simulink model "ProdSystem_BaseStockAssumptionsAndCosts"  (R2015a)
settings: Solver=ode45  SolverMode=SingleTasking  StartTime=0  StopTime=100000000  RelTol=1e-3
libraries: simeventslib x10, simulink x1
settings Model: CovSFcnEnable=off  Creator=AnotherUser  LastModifiedBy=gthiers3
settings OptimizationCC: BlockReduction=off  BooleanDataType=off
settings DebuggingCC: SaveWithParameterizedLinksMsg=none  UnderspecifiedInitializationDetection=Classic  MergeDetectMultiDrivingBlocksExec=none  SignalResolutionControl=TryResolveAllWithWarning
settings HardwareCC: TargetUnknown=on

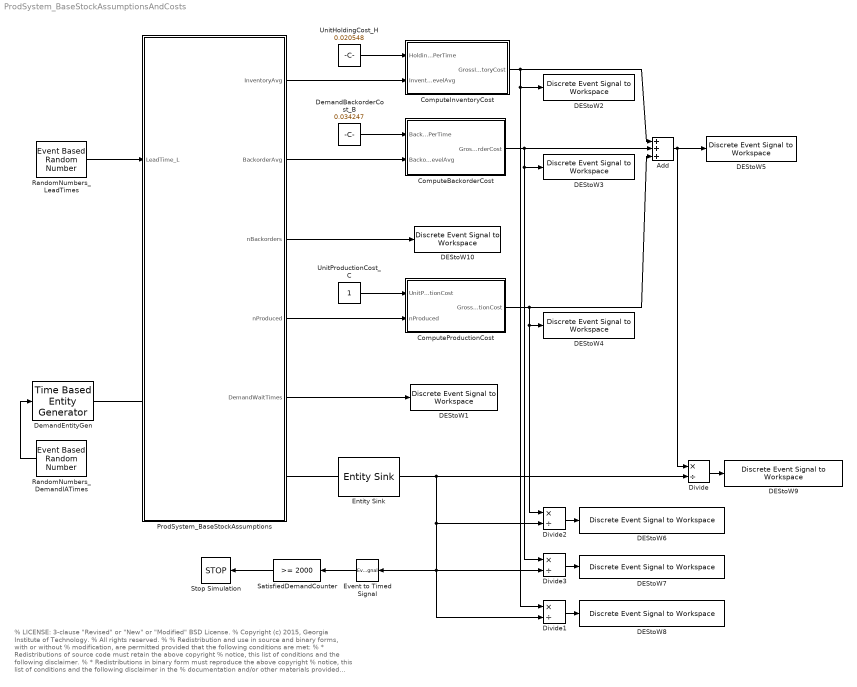
== system ProdSystem_BaseStockAssumptionsAndCosts ==
  note: % LICENSE: 3-clause "Revised" or "New" or "Modified" BSD License.
      | % Copyright (c) 2015, Georgia Institute of Technology.
      | % All rights reserved.
      | %
      | % Redistribution and use in source and binary forms, with or without
      | % modification, are permitted provided that the following conditions are met:
      | % * Redistributions of source code must retain the above copyright
      | % notice, this list of conditions and the following disclaimer.
      | % * Redistributions in binary form must reproduce the above copyright
      | % notice, this list of conditions and the following disclaimer in the
      | % documentation and/or other materials provided with the distribution.
      | % * Neither the name of the Georgia Institute of Technology nor the
      | % names of its contributors may be used to endorse or promote products
      | % derived from this software without specific prior written permission.
      | %
      | % THIS SOFTWARE IS PROVIDED BY THE COPYRIGHT HOLDERS AND CONTRIBUTORS "AS IS" AND
      | % ANY EXPRESS OR IMPLIED WARRANTIES, INCLUDING, BUT NOT LIMITED TO, THE IMPLIED
      | % WARRANTIES OF MERCHANTABILITY AND FITNESS FOR A PARTICULAR PURPOSE ARE
      | % DISCLAIMED. IN NO EVENT SHALL THE GEORGIA INSTITUTE OF TECHNOLOGY BE LIABLE FOR
      | % ANY DIRECT, INDIRECT, INCIDENTAL, SPECIAL, EXEMPLARY, OR CONSEQUENTIAL DAMAGES
      | % (INCLUDING, BUT NOT LIMITED TO, PROCUREMENT OF SUBSTITUTE GOODS OR SERVICES;
      | % LOSS OF USE, DATA, OR PROFITS; OR BUSINESS INTERRUPTION) HOWEVER CAUSED AND
      | % ON ANY THEORY OF LIABILITY, WHETHER IN CONTRACT, STRICT LIABILITY, OR TORT
      | % (INCLUDING NEGLIGENCE OR OTHERWISE) ARISING IN ANY WAY OUT OF THE USE OF THIS
      | % SOFTWARE, EVEN IF ADVISED OF THE POSSIBILITY OF SUCH DAMAGE.
  Add : Sum  Inputs=+++
  ComputeBackorderCost : Subsystem
  ComputeInventoryCost : Subsystem
  ComputeProductionCost : Subsystem
  DEStoW1 : simeventslib/SimEvents Sinks/Discrete Event Signal to Workspace  VariableName=DemandWaitTimes  SaveFormat=Structure With Time  isMonitorOnly=off  isRecordIC=off
  DEStoW10 : simeventslib/SimEvents Sinks/Discrete Event Signal to Workspace  VariableName=nBackorders  SaveFormat=Structure With Time  isMonitorOnly=off  isRecordIC=off
  DEStoW2 : simeventslib/SimEvents Sinks/Discrete Event Signal to Workspace  VariableName=GrossInventoryCost  SaveFormat=Structure With Time  isMonitorOnly=off  isRecordIC=off
  DEStoW3 : simeventslib/SimEvents Sinks/Discrete Event Signal to Workspace  VariableName=GrossBackorderCost  SaveFormat=Structure With Time  isMonitorOnly=off  isRecordIC=off
  DEStoW4 : simeventslib/SimEvents Sinks/Discrete Event Signal to Workspace  VariableName=GrossProductionCost  SaveFormat=Structure With Time  isMonitorOnly=off  isRecordIC=off
  DEStoW5 : simeventslib/SimEvents Sinks/Discrete Event Signal to Workspace  VariableName=GrossCost  SaveFormat=Structure With Time  isMonitorOnly=off  isRecordIC=off
  DEStoW6 : simeventslib/SimEvents Sinks/Discrete Event Signal to Workspace  VariableName=GrossProductionCost_PerSatDmd  SaveFormat=Structure With Time  isMonitorOnly=off  isRecordIC=off
  DEStoW7 : simeventslib/SimEvents Sinks/Discrete Event Signal to Workspace  VariableName=GrossBackorderCost_PerSatDmd  SaveFormat=Structure With Time  isMonitorOnly=off  isRecordIC=off
  DEStoW8 : simeventslib/SimEvents Sinks/Discrete Event Signal to Workspace  VariableName=GrossInventoryCost_PerSatDmd  SaveFormat=Structure With Time  isMonitorOnly=off  isRecordIC=off
  DEStoW9 : simeventslib/SimEvents Sinks/Discrete Event Signal to Workspace  VariableName=GrossCost_PerSatDmd  SaveFormat=Structure With Time  isMonitorOnly=off  isRecordIC=off
  DemandBackorderCost_B : Constant  Value=0.034247
  DemandEntityGen : TimeBasedEntityGenerator  GenerateEntitiesUpon=Intergeneration time from port t  GenerateEntityAtSimulationStart=off
  Divide{,1..3} (4 alike) : Product  Inputs=*/
  Entity Sink : EntitySink  StatNumberArrived=on
  Event to Timed Signal : EventToTimedSignal
  ProdSystem_BaseStockAssumptions : Subsystem  mask{BaseStockLevel=11}
      mask prompts: BaseStockLevel "Base Stock Level R:"
      mask TypeOptions BaseStockLevel: FcnCallGen_T0/NumberOfEventsPerPeriod
      mask DialogControl DescTextVar Prompt: (1) Demands occur randomly and one at a time, (2) Demand which is not filled immediately is backordered, (3) Replenishment lead times are known and deterministic (relaxed here - they can be random, or deterministic by choosing the normal distribution with stdev=eps, which is as close to zero as possible), (4) A replenishment order for a single unit is placed each time a demand occurs, and there is no constraint on the number of such orders.
  RandomNumbers_DemandIATimes : EventBasedRandomNumber  Distribution=Gamma  meanExp=8.76  scaleGam=73  meanNorm=73  stdNorm=73  scaleLogn=3.9439  shapeLogn=0.83255  Seed=32404
  RandomNumbers_LeadTimes : EventBasedRandomNumber  Distribution=Gamma  meanExp=8.76  scaleGam=1460  shapeGam=0.5  meanNorm=730  stdNorm=0.00013053  scaleLogn=6.593  shapeLogn=1.7881e-07  Seed=35621
  SatisfiedDemandCounter : simulink/Logic and Bit Operations/Compare To Constant  relop=>=  const=2000  OutDataTypeStr=boolean
  Stop Simulation : Stop
  UnitHoldingCost_H : Constant  Value=0.020548
  UnitProductionCost_C : Constant
  wires:
  RandomNumbers_DemandIATimes/1 -> DemandEntityGen/1
  Add/1 -> DEStoW5/1, Divide/1
  ProdSystem_BaseStockAssumptions/5(DemandWaitTimes) -> DEStoW1/1
  Divide/1 -> DEStoW9/1
  Divide1/1 -> DEStoW8/1
  Divide2/1 -> DEStoW6/1
  Divide3/1 -> DEStoW7/1
  RandomNumbers_LeadTimes/1 -> ProdSystem_BaseStockAssumptions/1(LeadTime_L)
  ComputeInventoryCost/1(GrossInventoryCost) -> Divide1/1, DEStoW2/1, Add/1
  UnitHoldingCost_H/1 -> ComputeInventoryCost/1(HoldingCost_PerUnitPerTime)
  ProdSystem_BaseStockAssumptions/1(InventoryAvg) -> ComputeInventoryCost/2(InventoryLevelAvg)
  ComputeBackorderCost/1(GrossBackorderCost) -> DEStoW3/1, Divide3/1, Add/2
  ProdSystem_BaseStockAssumptions/2(BackorderAvg) -> ComputeBackorderCost/2(BackorderLevelAvg)
  DemandBackorderCost_B/1 -> ComputeBackorderCost/1(BackorderCost_PerUnitPerTime)
  ComputeProductionCost/1(GrossProductionCost) -> Add/3, DEStoW4/1, Divide2/1
  ProdSystem_BaseStockAssumptions/4(nProduced) -> ComputeProductionCost/2(nProduced)
  UnitProductionCost_C/1 -> ComputeProductionCost/1(UnitProductionCost)
  ProdSystem_BaseStockAssumptions/3(nBackorders) -> DEStoW10/1
  Entity Sink/1 -> Divide3/2, Event to Timed Signal/1, Divide1/2, Divide2/2, Divide/2
  Event to Timed Signal/1 -> SatisfiedDemandCounter/1
  SatisfiedDemandCounter/1 -> Stop Simulation/1
  connections:
  DemandEntityGen/RConn1 -- ProdSystem_BaseStockAssumptions/LConn1
  ProdSystem_BaseStockAssumptions/RConn1 -- Entity Sink/LConn1

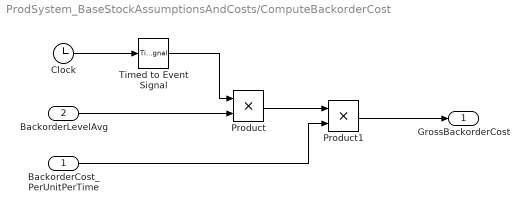
== system ProdSystem_BaseStockAssumptionsAndCosts/ComputeBackorderCost ==
  BackorderCost_PerUnitPerTime : Inport
  BackorderLevelAvg : Inport  Port=2
  Clock : Clock
  Product : Product
  Product1 : Product
  Timed to Event Signal : TimedToEventSignal
  GrossBackorderCost : Outport
  wires:
  BackorderLevelAvg/1 -> Product/2
  Product/1 -> Product1/1
  BackorderCost_PerUnitPerTime/1 -> Product1/2
  Product1/1 -> GrossBackorderCost/1
  Clock/1 -> Timed to Event Signal/1
  Timed to Event Signal/1 -> Product/1

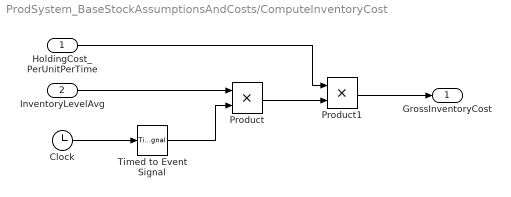
== system ProdSystem_BaseStockAssumptionsAndCosts/ComputeInventoryCost ==
  HoldingCost_PerUnitPerTime : Inport
  InventoryLevelAvg : Inport  Port=2
  Clock : Clock
  Product : Product
  Product1 : Product
  Timed to Event Signal : TimedToEventSignal
  GrossInventoryCost : Outport
  wires:
  Clock/1 -> Timed to Event Signal/1
  Timed to Event Signal/1 -> Product/2
  InventoryLevelAvg/1 -> Product/1
  Product/1 -> Product1/2
  HoldingCost_PerUnitPerTime/1 -> Product1/1
  Product1/1 -> GrossInventoryCost/1

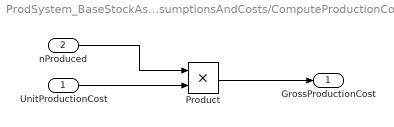
== system ProdSystem_BaseStockAssumptionsAndCosts/ComputeProductionCost ==
  UnitProductionCost : Inport
  nProduced : Inport  Port=2
  Product : Product
  GrossProductionCost : Outport
  wires:
  nProduced/1 -> Product/1
  UnitProductionCost/1 -> Product/2
  Product/1 -> GrossProductionCost/1

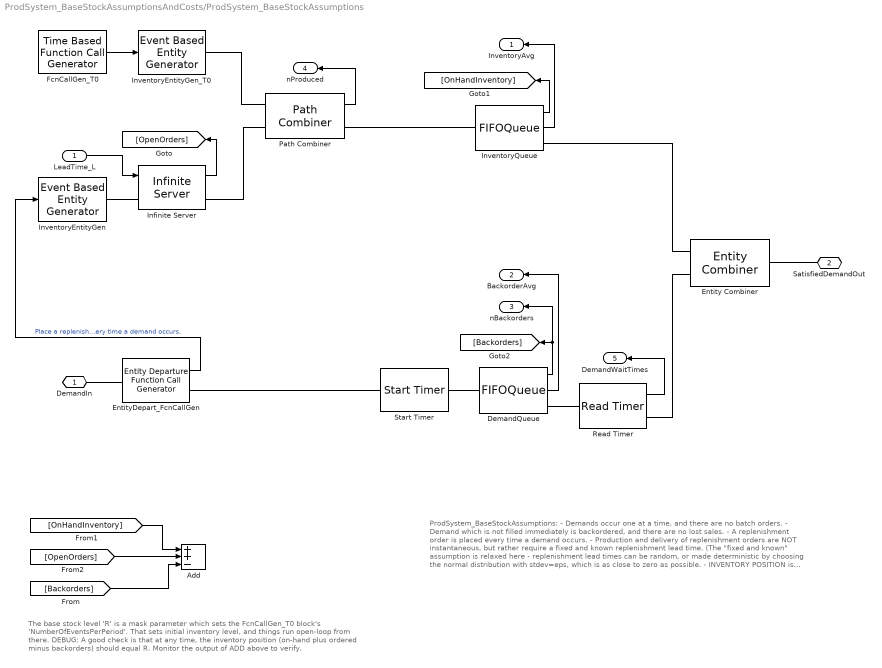
== system ProdSystem_BaseStockAssumptionsAndCosts/ProdSystem_BaseStockAssumptions ==
  note: The base stock level 'R' is a mask parameter which sets
      | the FcnCallGen_T0 block's 'NumberOfEventsPerPeriod'.
      | That sets initial inventory level, and things run open-loop
      | from there.
      |
      | DEBUG: A good check is that at any time, the inventory
      | position (on-hand plus ordered minus backorders) should
      | equal R. Monitor the output of ADD above to verify.
  note: ProdSystem_BaseStockAssumptions:
      |
      | - Demands occur one at a time, and there are no batch orders.
      |
      | - Demand which is not filled immediately is backordered, and there are no lost sales.
      |
      | - A replenishment order is placed every time a demand occurs.
      |
      | - Production and delivery of replenishment orders are NOT instantaneous, but rather require a
      | fixed and known replenishment lead time. (The "fixed and known" assumption is relaxed here -
      | replenishment lead times can be random, or made deterministic by choosing the normal
      | distribution with stdev=eps, which is as close to zero as possible.
      |
      | - INVENTORY POSITION is defined as on-hand inventory, plus open orders (not yet filled due to
      | replenishment lead time), minus backorders. The inventory position should always equal the
      | base stock level R.
  LeadTime_L : Inport
  Add : Sum  Inputs=++-
  DemandQueue : FIFOQueue  Capacity=Inf  StatNumberInBlock=on  StatAverageQueueLength=on
      settings: OutputPortMap=o1,o3
  Entity Combiner : EntityCombiner  NumberInputPorts=2  AttributeAccessibility=off  TimerAccessibility=off
  EntityDepart_FcnCallGen : EntityDepartureFunctionCallGenerator
  FcnCallGen_T0 : TimeBasedFunctionCallGenerator  EventGenerationMode=Only at simulation start  NumberOfEventsPerPeriod=BaseStockLevel
  Infinite Server : InfiniteServer  ServiceTimeFrom=Signal port t  StatNumberInBlock=on
      settings: OutputPortMap=o1
  InventoryEntityGen : EventBasedEntityGenerator  GenerateEntitiesUpon=Function call from port fcn
  InventoryEntityGen_T0 : EventBasedEntityGenerator  GenerateEntitiesUpon=Function call from port fcn
  InventoryQueue : FIFOQueue  Capacity=Inf  StatNumberInBlock=on  StatAverageQueueLength=on
      settings: OutputPortMap=o1,o3
  Path Combiner : PathCombiner  NumberInputPorts=2  StatNumberDeparted=on
  Read Timer : ReadTimer  StatTimeElapsed=on
      settings: OutputPortMap=o2
  Start Timer : StartTimer
  DemandIn : PMIOPort  Port=1  Side=Left
  SatisfiedDemandOut : PMIOPort  Port=2  Side=Right
  InventoryAvg : Outport
  BackorderAvg : Outport  Port=2
  nBackorders : Outport  Port=3
  nProduced : Outport  Port=4
  DemandWaitTimes : Outport  Port=5
  wires:
  LeadTime_L/1 -> Infinite Server/1
  EntityDepart_FcnCallGen/1 -> InventoryEntityGen/1  "Place a replenishment order every time a demand occurs."
  FcnCallGen_T0/1 -> InventoryEntityGen_T0/1
  DemandQueue/2 -> BackorderAvg/1
  Path Combiner/1 -> nProduced/1
  Read Timer/1 -> DemandWaitTimes/1
  InventoryQueue/2 -> InventoryAvg/1
  Infinite Server/1 -> [OpenOrders]
  InventoryQueue/1 -> [OnHandInventory]
  DemandQueue/1 -> nBackorders/1, [Backorders]
  [OpenOrders] -> Add/2
  [OnHandInventory] -> Add/1
  [Backorders] -> Add/3
  connections:
  Read Timer/RConn1 -- Entity Combiner/LConn2
  Entity Combiner/RConn1 -- SatisfiedDemandOut/RConn1
  InventoryEntityGen/RConn1 -- Infinite Server/LConn1
  InventoryQueue/LConn1 -- Path Combiner/RConn1
  DemandQueue/LConn1 -- Start Timer/RConn1
  DemandQueue/RConn1 -- Read Timer/LConn1
  DemandIn/RConn1 -- EntityDepart_FcnCallGen/LConn1
  EntityDepart_FcnCallGen/RConn1 -- Start Timer/LConn1
  InventoryEntityGen_T0/RConn1 -- Path Combiner/LConn1
  Infinite Server/RConn1 -- Path Combiner/LConn2
  InventoryQueue/RConn1 -- Entity Combiner/LConn1
